simulink model "Point_Kinetic"  (R2023a)
settings: Solver=VariableStepAuto  StartTime=0.0  StopTime=10.0  RelTol=1e-3
settings Model: Creator=bulldize  LastModifiedBy=bulldize

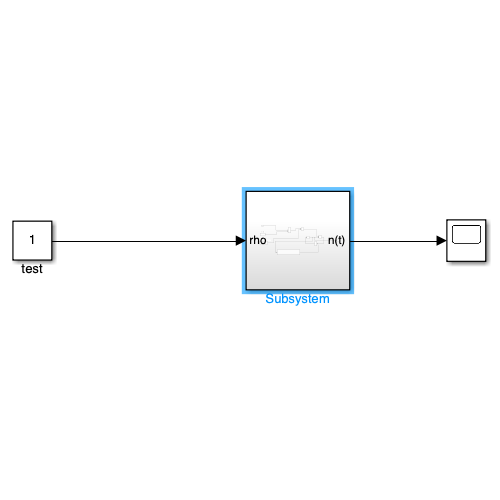
[thumbnail: Simulink's stored preview of the top-level diagram]
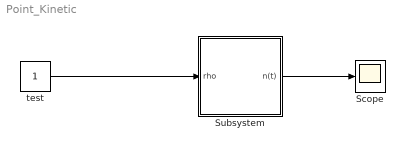
== system Point_Kinetic ==
  Scope : Scope
  Subsystem : Subsystem
  test : Constant
  wires:
  test/1 -> Subsystem/1(rho)
  Subsystem/1(n(t)) -> Scope/1

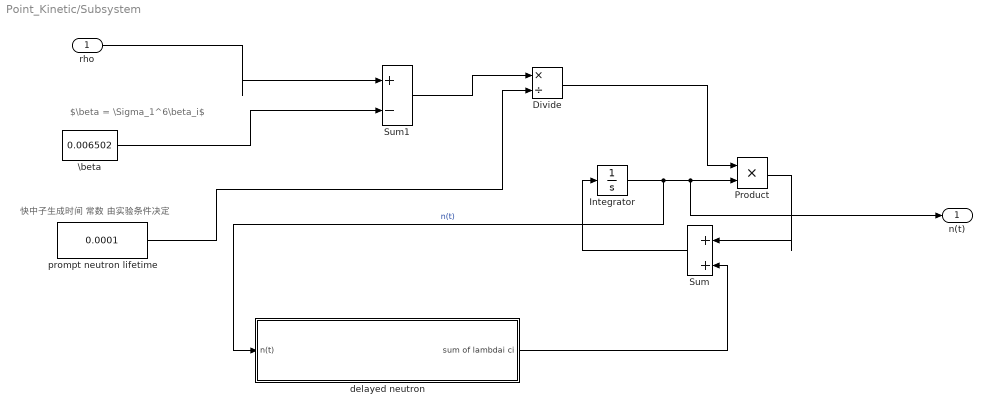
== system Point_Kinetic/Subsystem ==
  note: $\beta = \Sigma_1^6\beta_i$
  note: 快中子生成时间 常数 由实验条件决定
  rho : Inport
  Divide : Product  Inputs=*/
  Integrator : Integrator  InitialCondition=0.05
  Product : Product
  Sum : Sum  Inputs=|++
  Sum1 : Sum  Inputs=|+-
  \beta : Constant  Value=0.006502
  delayed neutron : Subsystem
  prompt neutron lifetime : Constant  Value=0.0001
  n(t) : Outport
  wires:
  Integrator/1 -> delayed neutron/1(n(t)), n(t)/1, Product/2  "n(t)"
  rho/1 -> Sum1/1
  \beta/1 -> Sum1/2
  Sum1/1 -> Divide/1
  prompt neutron lifetime/1 -> Divide/2
  Divide/1 -> Product/1
  Product/1 -> Sum/1
  delayed neutron/1(sum of lambdai ci) -> Sum/2
  Sum/1 -> Integrator/1

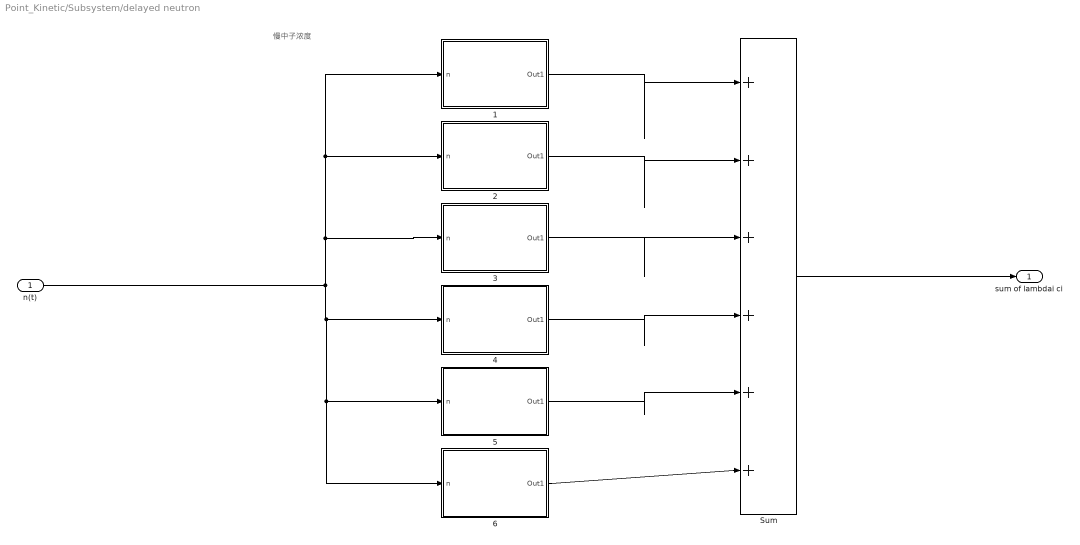
== system Point_Kinetic/Subsystem/delayed neutron ==
  note: 慢中子浓度
  n(t) : Inport
  1 : Subsystem
  2 : Subsystem
  3 : Subsystem
  4 : Subsystem
  5 : Subsystem
  6 : Subsystem
  Sum : Sum  Inputs=|++++++
  sum of lambdai ci : Outport
  wires:
  3/1(Out1) -> Sum/3
  1/1(Out1) -> Sum/1
  6/1(Out1) -> Sum/6
  4/1(Out1) -> Sum/4
  2/1(Out1) -> Sum/2
  Sum/1 -> sum of lambdai ci/1
  5/1(Out1) -> Sum/5
  n(t)/1 -> 3/1(n), 2/1(n), 1/1(n), 6/1(n), 5/1(n), 4/1(n)

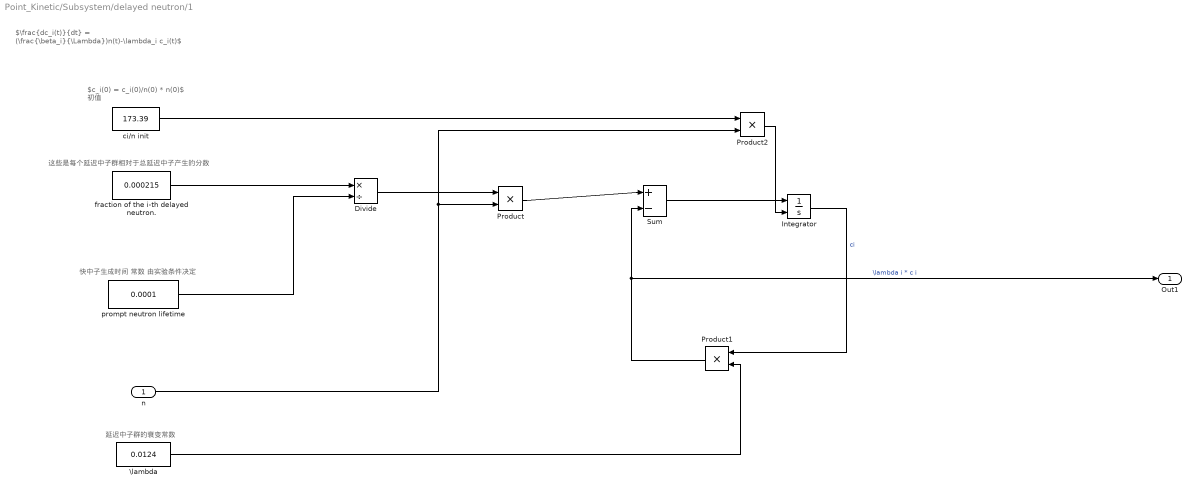
== system Point_Kinetic/Subsystem/delayed neutron/1 ==
  note: $c_i(0) = c_i(0)/n(0) * n(0)$ 初值
  note: 延迟中子群的衰变常数
  note: $\frac{dc_i(t)}{dt} = (\frac{\beta_i}{\Lambda})n(t)-\lambda_i c_i(t)$
  note: 这些是每个延迟中子群相对于总延迟中子产生的分数
  note: 快中子生成时间 常数 由实验条件决定
  n : Inport
  Divide : Product  Inputs=*/
  Integrator : Integrator  InitialConditionSource=external
  Product : Product
  Product1 : Product
  Product2 : Product
  Sum : Sum  Inputs=|+-
  \lambda : Constant  Value=0.0124
  ci/n init : Constant  Value=173.39
  fraction of the i-th delayed neutron. : Constant  Value=0.000215
  prompt neutron lifetime : Constant  Value=0.0001
  Out1 : Outport
  wires:
  fraction of the i-th delayed neutron./1 -> Divide/1
  prompt neutron lifetime/1 -> Divide/2
  Divide/1 -> Product/1
  n/1 -> Product2/2, Product/2
  Product/1 -> Sum/1
  Sum/1 -> Integrator/1
  \lambda/1 -> Product1/2
  Integrator/1 -> Product1/1  "ci"
  Product1/1 -> Out1/1, Sum/2  "\\lambda i * c i"
  ci/n init/1 -> Product2/1
  Product2/1 -> Integrator/2

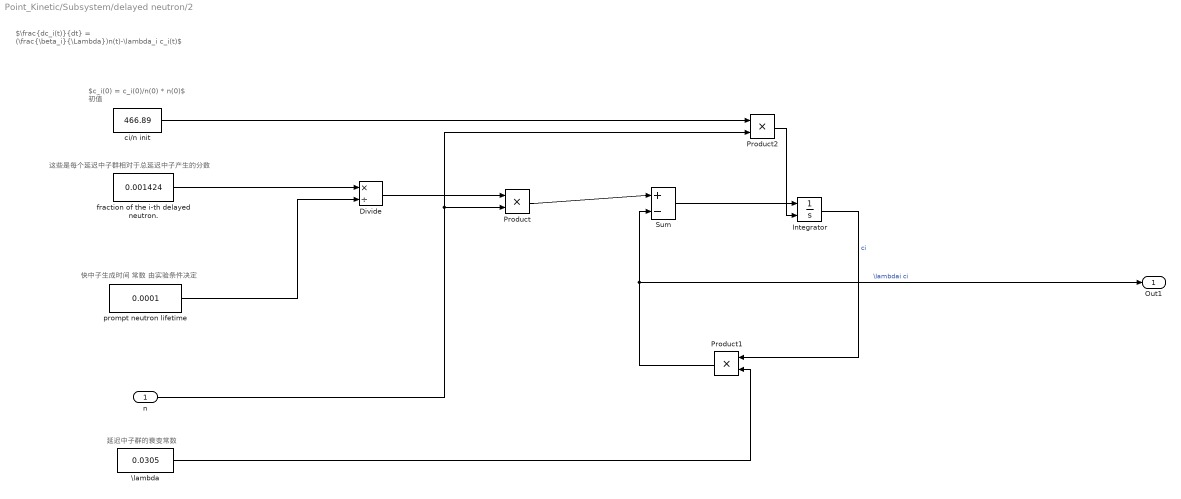
== system Point_Kinetic/Subsystem/delayed neutron/2 ==
  note: $c_i(0) = c_i(0)/n(0) * n(0)$ 初值
  note: 延迟中子群的衰变常数
  note: $\frac{dc_i(t)}{dt} = (\frac{\beta_i}{\Lambda})n(t)-\lambda_i c_i(t)$
  note: 这些是每个延迟中子群相对于总延迟中子产生的分数
  note: 快中子生成时间 常数 由实验条件决定
  n : Inport
  Divide : Product  Inputs=*/
  Integrator : Integrator  InitialConditionSource=external
  Product : Product
  Product1 : Product
  Product2 : Product
  Sum : Sum  Inputs=|+-
  \lambda : Constant  Value=0.0305
  ci/n init : Constant  Value=466.89
  fraction of the i-th delayed neutron. : Constant  Value=0.001424
  prompt neutron lifetime : Constant  Value=0.0001
  Out1 : Outport
  wires:
  fraction of the i-th delayed neutron./1 -> Divide/1
  prompt neutron lifetime/1 -> Divide/2
  Divide/1 -> Product/1
  n/1 -> Product2/2, Product/2
  Product/1 -> Sum/1
  Sum/1 -> Integrator/1
  \lambda/1 -> Product1/2
  Integrator/1 -> Product1/1  "ci"
  Product1/1 -> Out1/1, Sum/2  "\\lambdai ci"
  ci/n init/1 -> Product2/1
  Product2/1 -> Integrator/2

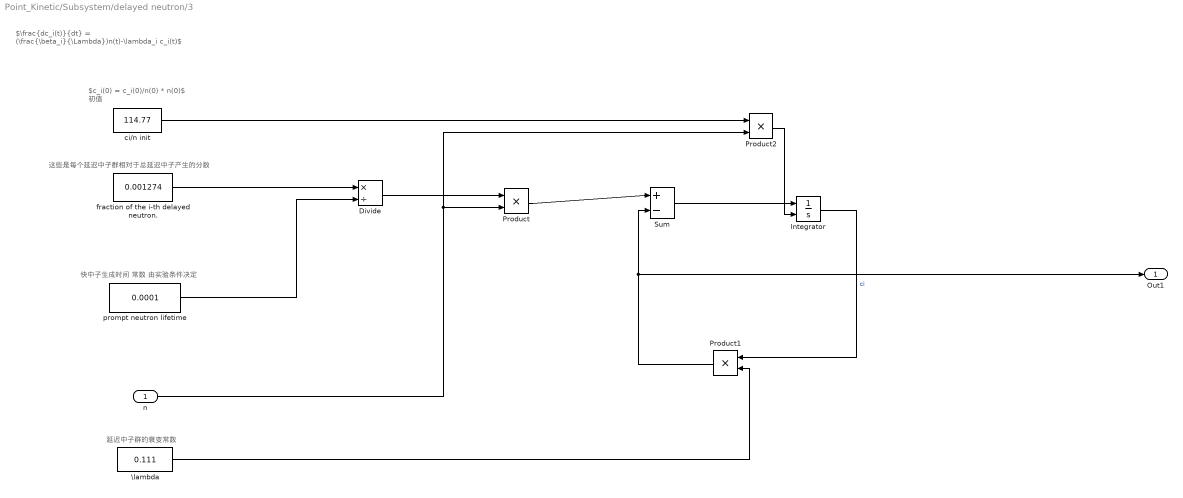
== system Point_Kinetic/Subsystem/delayed neutron/3 ==
  note: $c_i(0) = c_i(0)/n(0) * n(0)$ 初值
  note: 延迟中子群的衰变常数
  note: $\frac{dc_i(t)}{dt} = (\frac{\beta_i}{\Lambda})n(t)-\lambda_i c_i(t)$
  note: 这些是每个延迟中子群相对于总延迟中子产生的分数
  note: 快中子生成时间 常数 由实验条件决定
  n : Inport
  Divide : Product  Inputs=*/
  Integrator : Integrator  InitialConditionSource=external
  Product : Product
  Product1 : Product
  Product2 : Product
  Sum : Sum  Inputs=|+-
  \lambda : Constant  Value=0.111
  ci/n init : Constant  Value=114.77
  fraction of the i-th delayed neutron. : Constant  Value=0.001274
  prompt neutron lifetime : Constant  Value=0.0001
  Out1 : Outport
  wires:
  fraction of the i-th delayed neutron./1 -> Divide/1
  prompt neutron lifetime/1 -> Divide/2
  Divide/1 -> Product/1
  n/1 -> Product2/2, Product/2
  Product/1 -> Sum/1
  Sum/1 -> Integrator/1
  \lambda/1 -> Product1/2
  Integrator/1 -> Product1/1  "ci"
  Product1/1 -> Sum/2, Out1/1
  ci/n init/1 -> Product2/1
  Product2/1 -> Integrator/2

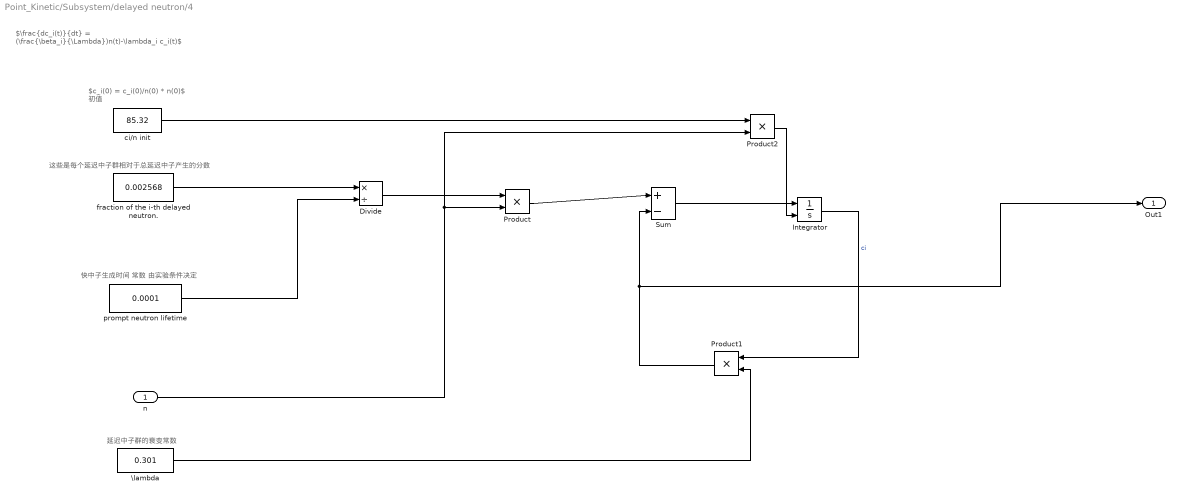
== system Point_Kinetic/Subsystem/delayed neutron/4 ==
  note: $c_i(0) = c_i(0)/n(0) * n(0)$ 初值
  note: 延迟中子群的衰变常数
  note: $\frac{dc_i(t)}{dt} = (\frac{\beta_i}{\Lambda})n(t)-\lambda_i c_i(t)$
  note: 这些是每个延迟中子群相对于总延迟中子产生的分数
  note: 快中子生成时间 常数 由实验条件决定
  n : Inport
  Divide : Product  Inputs=*/
  Integrator : Integrator  InitialConditionSource=external
  Product : Product
  Product1 : Product
  Product2 : Product
  Sum : Sum  Inputs=|+-
  \lambda : Constant  Value=0.301
  ci/n init : Constant  Value=85.32
  fraction of the i-th delayed neutron. : Constant  Value=0.002568
  prompt neutron lifetime : Constant  Value=0.0001
  Out1 : Outport
  wires:
  fraction of the i-th delayed neutron./1 -> Divide/1
  prompt neutron lifetime/1 -> Divide/2
  Divide/1 -> Product/1
  n/1 -> Product2/2, Product/2
  Product/1 -> Sum/1
  Sum/1 -> Integrator/1
  \lambda/1 -> Product1/2
  Integrator/1 -> Product1/1  "ci"
  Product1/1 -> Out1/1, Sum/2
  ci/n init/1 -> Product2/1
  Product2/1 -> Integrator/2

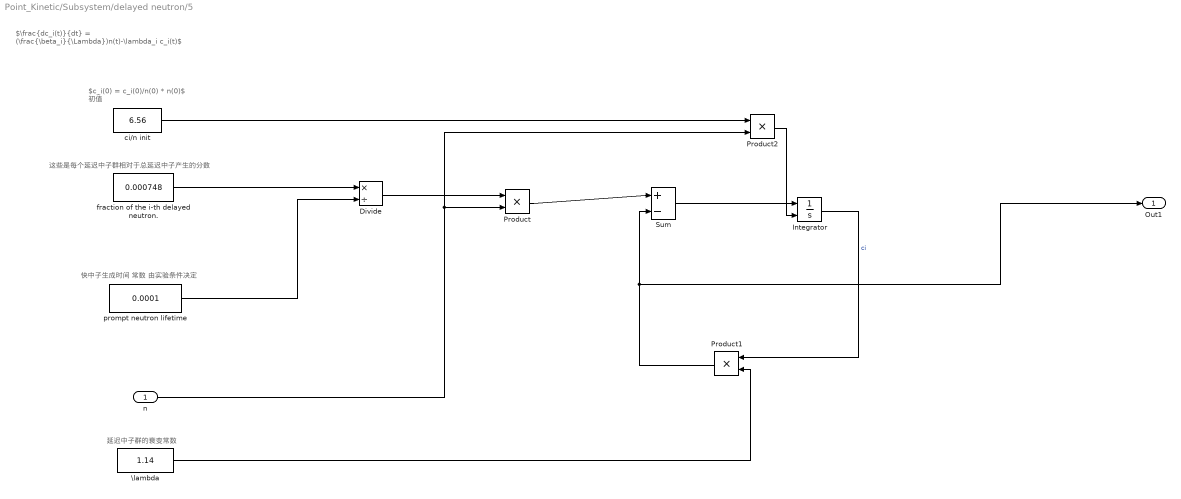
== system Point_Kinetic/Subsystem/delayed neutron/5 ==
  note: $c_i(0) = c_i(0)/n(0) * n(0)$ 初值
  note: 延迟中子群的衰变常数
  note: $\frac{dc_i(t)}{dt} = (\frac{\beta_i}{\Lambda})n(t)-\lambda_i c_i(t)$
  note: 这些是每个延迟中子群相对于总延迟中子产生的分数
  note: 快中子生成时间 常数 由实验条件决定
  n : Inport
  Divide : Product  Inputs=*/
  Integrator : Integrator  InitialConditionSource=external
  Product : Product
  Product1 : Product
  Product2 : Product
  Sum : Sum  Inputs=|+-
  \lambda : Constant  Value=1.14
  ci/n init : Constant  Value=6.56
  fraction of the i-th delayed neutron. : Constant  Value=0.000748
  prompt neutron lifetime : Constant  Value=0.0001
  Out1 : Outport
  wires:
  fraction of the i-th delayed neutron./1 -> Divide/1
  prompt neutron lifetime/1 -> Divide/2
  Divide/1 -> Product/1
  n/1 -> Product2/2, Product/2
  Product/1 -> Sum/1
  Sum/1 -> Integrator/1
  \lambda/1 -> Product1/2
  Integrator/1 -> Product1/1  "ci"
  Product1/1 -> Out1/1, Sum/2
  ci/n init/1 -> Product2/1
  Product2/1 -> Integrator/2

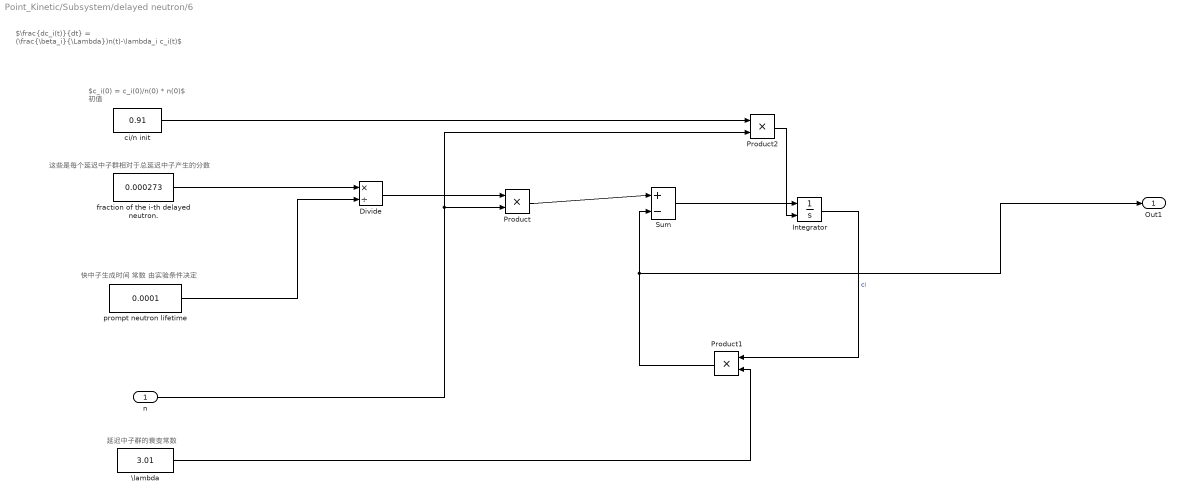
== system Point_Kinetic/Subsystem/delayed neutron/6 ==
  note: $c_i(0) = c_i(0)/n(0) * n(0)$ 初值
  note: 延迟中子群的衰变常数
  note: $\frac{dc_i(t)}{dt} = (\frac{\beta_i}{\Lambda})n(t)-\lambda_i c_i(t)$
  note: 这些是每个延迟中子群相对于总延迟中子产生的分数
  note: 快中子生成时间 常数 由实验条件决定
  n : Inport
  Divide : Product  Inputs=*/
  Integrator : Integrator  InitialConditionSource=external
  Product : Product
  Product1 : Product
  Product2 : Product
  Sum : Sum  Inputs=|+-
  \lambda : Constant  Value=3.01
  ci/n init : Constant  Value=0.91
  fraction of the i-th delayed neutron. : Constant  Value=0.000273
  prompt neutron lifetime : Constant  Value=0.0001
  Out1 : Outport
  wires:
  fraction of the i-th delayed neutron./1 -> Divide/1
  prompt neutron lifetime/1 -> Divide/2
  Divide/1 -> Product/1
  n/1 -> Product2/2, Product/2
  Product/1 -> Sum/1
  Sum/1 -> Integrator/1
  \lambda/1 -> Product1/2
  Integrator/1 -> Product1/1  "ci"
  Product1/1 -> Out1/1, Sum/2
  ci/n init/1 -> Product2/1
  Product2/1 -> Integrator/2
